simulink model "zad1"  (R2022b)
settings: Solver=VariableStepAuto  StartTime=0.0  StopTime=10.0  RelTol=1e-3
settings Model: Creator=maciejholodniuk  LastModifiedBy=maciejholodniuk

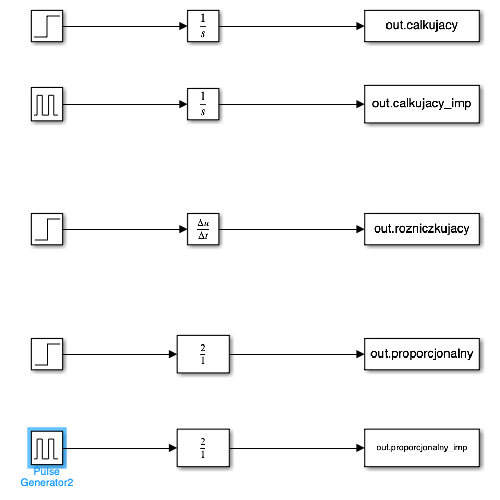
[thumbnail: Simulink's stored preview of the top-level diagram]
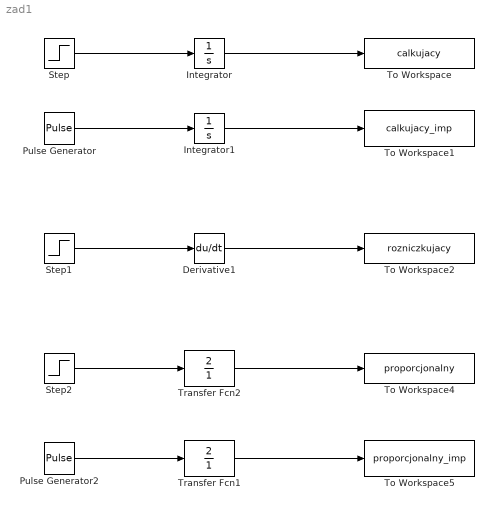
== system zad1 ==
  Derivative1 : Derivative
  Integrator : Integrator
  Integrator1 : Integrator
  Pulse Generator : DiscretePulseGenerator  PulseType=Time based  Amplitude=20  Period=10  PulseWidth=0.5  PhaseDelay=1
  Pulse Generator2 : DiscretePulseGenerator  PulseType=Time based  Period=10  PulseWidth=0.5  PhaseDelay=1
  Step : Step  SampleTime=0
  Step1 : Step  SampleTime=0
  Step2 : Step  SampleTime=0
  To Workspace : ToWorkspace  VariableName=calkujacy  SaveFormat=Timeseries  SampleTime=-1
  To Workspace1 : ToWorkspace  VariableName=calkujacy_imp  SaveFormat=Timeseries  SampleTime=-1
  To Workspace2 : ToWorkspace  VariableName=rozniczkujacy  SaveFormat=Timeseries  SampleTime=-1
  To Workspace4 : ToWorkspace  VariableName=proporcjonalny  SaveFormat=Timeseries  SampleTime=-1
  To Workspace5 : ToWorkspace  VariableName=proporcjonalny_imp  SaveFormat=Timeseries  SampleTime=-1
  Transfer Fcn1 : TransferFcn  Numerator=[0 2]  Denominator=[0 1]
  Transfer Fcn2 : TransferFcn  Numerator=[0 2]  Denominator=[0 1]
  wires:
  Step/1 -> Integrator/1
  Integrator/1 -> To Workspace/1
  Integrator1/1 -> To Workspace1/1
  Pulse Generator/1 -> Integrator1/1
  Step1/1 -> Derivative1/1
  Derivative1/1 -> To Workspace2/1
  Step2/1 -> Transfer Fcn2/1
  Transfer Fcn2/1 -> To Workspace4/1
  Pulse Generator2/1 -> Transfer Fcn1/1
  Transfer Fcn1/1 -> To Workspace5/1
